simulink model "LinkLabelEmpty.multi"  (R2014b)
settings: Solver=ode45  StartTime=0.0  StopTime=10.0  RelTol=1e-3
settings Model: Creator=tkr5kor  LastModifiedBy=tkr5kor

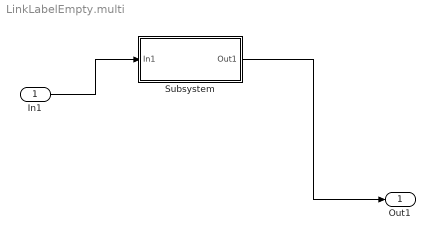
== system LinkLabelEmpty.multi ==
  In1 : Inport
  Subsystem : Subsystem
  Out1 : Outport
  wires:
  In1/1 -> Subsystem/1(In1)
  Subsystem/1(Out1) -> Out1/1

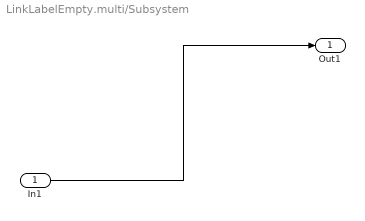
== system LinkLabelEmpty.multi/Subsystem ==
  In1 : Inport
  Out1 : Outport
  wires:
  In1/1 -> Out1/1
